simulink model "wifiBPara"  (R2022a)
settings: Solver=ode5  StartTime=0.0  StopTime=simuSpan  FixedStep=Ts  RelTol=1e-3  EnableMultiTasking=on
values from neighbouring files (symbols this model uses):
  bbSymRate = symRate*11    [wifiB4IFPLL.m]
  fifEst = 2.006e8    (= 200600000)    [PLLLockDebug.m]    (also in wifiB3IFGen.m)
  Ts = 1/fs    (= 5e-11)    [wifiB00main.m]
libraries: dsparch4 x3, dspxfrm3 x1, commsynccomp2 x1
settings Model: Creator=adminYuan  LastModifiedBy=adminYuan
settings DataIOCC: LimitDataPoints=on  SaveFormat=Array  SignalLoggingSaveFormat=ModelDataLogs  ReturnWorkspaceOutputs=off  SignalLoggingName=sigsOut
settings OptimizationCC: InitFltsAndDblsToZero=on  LifeSpan=inf
settings DebuggingCC: SaveWithParameterizedLinksMsg=none  UnderspecifiedInitializationDetection=Classic  MergeDetectMultiDrivingBlocksExec=none  SignalResolutionControl=TryResolveAllWithWarning  MultiTaskDSMMsg=warning  MultiTaskCondExecSysMsg=none  UnconnectedInputMsg=warning  UnconnectedOutputMsg=warning  UnconnectedLineMsg=warning  SFUnexpectedBacktrackingDiag=warning  SFNoUnconditionalDefaultTransitionDiag=warning  SFExecutionAtInitializationDiag=none  SFMachineParentedDataDiag=warning  ArithmeticOperatorsInVariantConditions=warning
settings HardwareCC: ProdBitPerPointer=32  ProdBitPerSizeT=32  ProdBitPerPtrDiffT=32  ProdLargestAtomicFloat=None  ProdIntDivRoundTo=Undefined  ProdEndianess=Unspecified  ProdWordSize=32  ProdHWDeviceType=32-bit Generic  TargetUnknown=on
settings ModelReferenceCC: PropagateSignalLabelsOutOfModel=off
settings CodeAppCC: StateflowObjectComments=on
settings GRTTargetCC: TargetFcnLib=ansi_tfl_tmw.mat  TargetLangStandard=C89/C90 (ANSI)  CombineOutputUpdateFcns=off  GRTInterface=on
settings ConfigComp: CovMetricSettings=dw  CovSaveCumulativeToWorkspaceVar=on  CovSaveSingleToWorkspaceVar=on

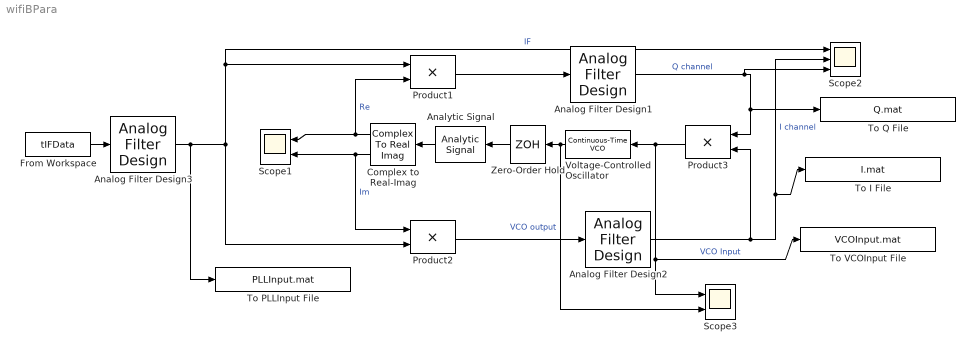
== system wifiBPara ==
  Analog Filter Design1 : dsparch4/Analog Filter Design  method=Butterworth  filttype=Lowpass  N=6  Wlo=2*pi*bbSymRate*10  Whi=2*pi*22e3  Rp=2  Rs=40
  Analog Filter Design2 : dsparch4/Analog Filter Design  method=Butterworth  filttype=Lowpass  N=6  Wlo=2*pi*bbSymRate*10  Whi=2*pi*22e3  Rp=2  Rs=40
  Analog Filter Design3 : dsparch4/Analog Filter Design  method=Butterworth  filttype=Bandpass  N=6  Wlo=2*pi*fifEst*(1/4)  Whi=2*pi*fifEst*(7/4)  Rp=2  Rs=40
  Analytic Signal : dspxfrm3/Analytic Signal  N=100  InputProcessing=Columns as channels (frame based)
      settings: SourceProductBaseCode=DS
  Complex to Real-Imag : ComplexToRealImag
  From Workspace : FromWorkspace  VariableName=tIFData  SampleTime=Ts  Interpolate=off  ZeroCross=off  OutputAfterFinalValue=Setting to zero
  Product1 : Product  SaturateOnIntegerOverflow=on  OutDataTypeStr=Inherit: Same as first input
  Product2 : Product  SaturateOnIntegerOverflow=on  OutDataTypeStr=Inherit: Same as first input
  Product3 : Product  SaturateOnIntegerOverflow=on  OutDataTypeStr=Inherit: Same as first input
  Scope1 : Scope  NumInputPorts=2
  Scope2 : Scope  NumInputPorts=3
  Scope3 : Scope  NumInputPorts=2
  To I File : ToFile  Filename=I.mat  MatrixName=I
  To PLLInput File : ToFile  Filename=PLLInput.mat  MatrixName=PLLInput
  To Q File : ToFile  Filename=Q.mat  MatrixName=Q
  To VCOInput File : ToFile  Filename=VCOInput.mat  MatrixName=VCOInput
  Voltage-Controlled Oscillator : commsynccomp2/Continuous-Time VCO  Ac=1  Fc=VCOQuiescentFre  Kc=VCOSensitivity  Ph=1
      settings: SourceProductBaseCode=CM
  Zero-Order Hold : ZeroOrderHold  SampleTime=Ts
  wires:
  Voltage-Controlled Oscillator/1 -> Zero-Order Hold/1, Scope3/2  "VCO output"
  Analytic Signal/1 -> Complex to Real-Imag/1
  Product1/1 -> Analog Filter Design1/1
  Product2/1 -> Analog Filter Design2/1
  Analog Filter Design1/1 -> Scope2/3, Product3/1, To Q File/1  "Q channel"
  Analog Filter Design2/1 -> Product3/2, To I File/1, Scope2/2  "I channel"
  Complex to Real-Imag/1 -> Product1/2, Scope1/1  "Re"
  Complex to Real-Imag/2 -> Product2/1, Scope1/2  "Im"
  Zero-Order Hold/1 -> Analytic Signal/1
  From Workspace/1 -> Analog Filter Design3/1
  Analog Filter Design3/1 -> Product2/2, Product1/1, Scope2/1, To PLLInput File/1  "IF"
  Product3/1 -> Voltage-Controlled Oscillator/1, Scope3/1, To VCOInput File/1  "VCO Input"
